simulink model "metodoT1"  (R2012b)
settings: Solver=ode45  StartTime=0.0  StopTime=1  RelTol=1e-3
libraries: BLDC x3, Encoder x2
settings Model: Creator=h3now  LastModifiedBy=h3now

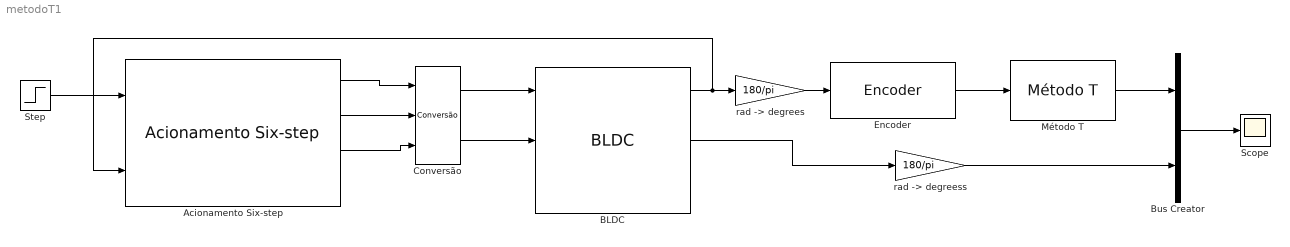
== system metodoT1 ==
  Acionamento Six-step : BLDC/Acionamento Six-step  P=8
  BLDC : BLDC/BLDC  J=1.39e-6  R=10.1/2  L=2.04/2000  P=8  Kt=15.7e-3/1.19  Ke=15.7e-3/1.19  Kd=0  F_stick=0  F_slip=0  default_fcem=on  fcem_a=fcem_a  fcem_b=fcem_b  fcem_c=fcem_c
  Bus Creator : BusCreator  Inputs=2
  Conversão : BLDC/Conversão
  Encoder : Encoder/Encoder  Nr=10
  Método T : Encoder/Método T  m=1
  Scope : Scope
      settings: YMin=12500  YMax=45000
  Step : Step  Time=0.31  Before=1  After=0  SampleTime=0
  "rad -> degrees" : Gain  Gain=180/pi
  "rad -> degreess" : Gain  Gain=180/pi
  wires:
  BLDC/2 -> "rad -> degreess"/1
  Bus Creator/1 -> Scope/1
  "rad -> degreess"/1 -> Bus Creator/2
  Encoder/1 -> Método T/1
  Método T/1 -> Bus Creator/1
  "rad -> degrees"/1 -> Encoder/1
  BLDC/1 -> Acionamento Six-step/2, "rad -> degrees"/1
  Conversão/2 -> BLDC/2
  Conversão/1 -> BLDC/1
  Acionamento Six-step/1 -> Conversão/1
  Acionamento Six-step/2 -> Conversão/2
  Acionamento Six-step/3 -> Conversão/3
  Step/1 -> Acionamento Six-step/1
